simulink model "tempest_bpsk"  (R2018b)
settings: Solver=FixedStepDiscrete  StartTime=0.0  StopTime=inf  RelTol=1e-3
undefined symbols (not defined in the file): designMultirateFIR
libraries: commrfcorlib x2, commsync2 x2, commsdrhw_v2 x1, dspmlti4 x1, dspsigops x1, commrflib2 x1, commfilt2 x1
settings Model: SimulationMode=accelerator  Creator=Joseph  LastModifiedBy=Joseph

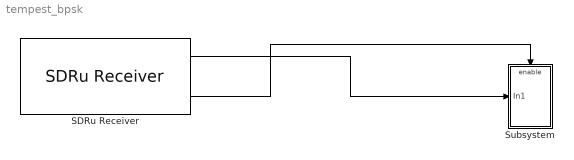
== system tempest_bpsk ==
  SDRu Receiver : commsdrhw_v2/SDRu Receiver  rxtx=rx  initializeIPAddress=0  devMap=0  USRP2_IP=192.168.10.2  USRP_IP_X300=192.168.10.2  USRP_IP_X310=192.168.10.2  USRP_serialNumB200=No devices found  USRP_serialNumB210=No devices found  platform=N200/N210/USRP2  prevPlatform=N200/N210/USRP2  lastIPAddressPopup=192.168.10.2  USRP_ID=192.168.10.2  LastIPAddress=192.168.10.2  ChannelMapping=1  centerFrequencySrc=Dialog  centerFrequency=54000000  loOffsetSrc=Dialog  loOffset=0  gainSrc=Dialog  gain=32  PPSSource=Internal  clockSource=Internal  masterClkRateParam=100e6  masterClkRateB200=32e6  masterClkRateB210=32e6  masterClkRateX300=200e6  masterClkRateX310=200e6  masterClkRate=100e6  decimInterpSrc=Dialog  decimInterp=512  USRP2_IP_NUM=[49 57 50 46 49 54 56 46 49 48 46 50]  TransportDataType=int16  overrunUnderrunPort=off  sampleTime=512/100e6  outputDatatype=double  frameLength=25472  HOST_DATA_PORT=0  HOST_CONTROL_PORT=0  USRP2_DATA_PORT=0  USRP2_CONTROL_PORT=0  bufferMode=Continuous streaming  EnableBurstMode=off  NumFramesInBurst=100
      settings: SourceProductName=Communications System Toolbox Support Package for USRP(R) Radio  SourceProductBaseCode=USRP
  Subsystem : Subsystem
  wires:
  SDRu Receiver/1 -> Subsystem/1(In1)
  SDRu Receiver/2 -> Subsystem/Enable

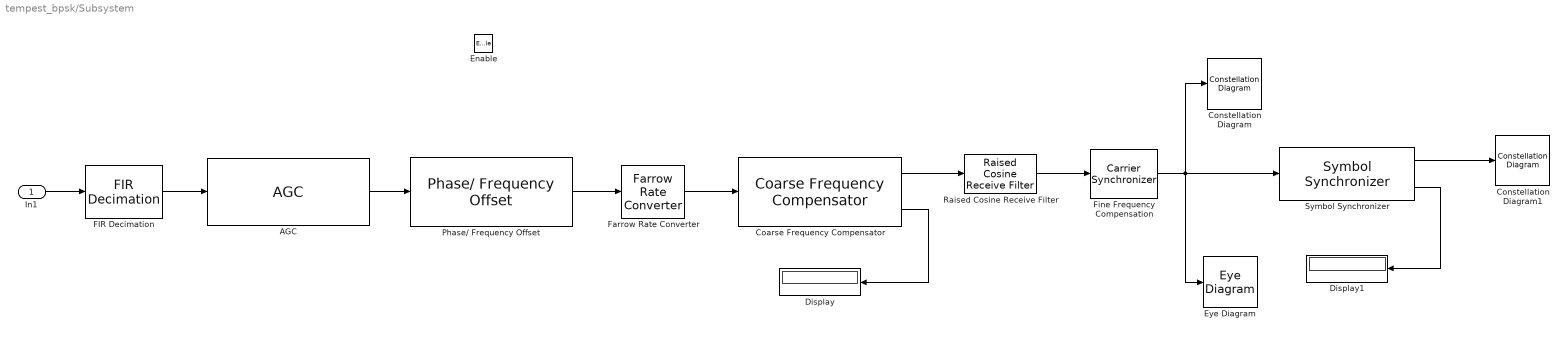
== system tempest_bpsk/Subsystem ==
  In1 : Inport
  Enable : EnablePort  PropagateVarSize=During execution
  AGC : commrfcorlib/AGC  LegacyMode=off  DetectorMethod=Rectifier  LoopMethod=Linear  UpdatePeriod=100  StepSize=0.1  AdaptationStepSize=0.01  DesiredOutputPower=1  AveragingLength=100  MaximumGain=30  MaxPowerGain=60  GainOutputPort=off  InputPowerOutputPort=off  SimulateUsing=Interpreted execution
      settings: SourceProductName=Communications System Toolbox
  Coarse Frequency Compensator : commrfcorlib/Coarse Frequency Compensator  Modulation=BPSK  Algorithm=FFT-based  FrequencyResolution=16  MaximumFrequencyOffset=3000  SamplesPerSymbol=4  EstimatedFreqOffsetPort=on  SimulateUsing=Code generation
      settings: SourceProductName=Communications System Toolbox  SourceProductBaseCode=CM
  Constellation Diagram : ConstellationDiagram
  Constellation Diagram1 : ConstellationDiagram
  Display : Display
      settings: Decimation=200
  Display1 : Display
      settings: Decimation=200
  Eye Diagram : EyeDiagram
  FIR Decimation : dspmlti4/FIR Decimation  FilterSource=Auto  h=designMultirateFIR(1,2)  D=16  filtStruct=Direct form  FilterObject=FDECIM  InputProcessing=Columns as channels (frame based)  framing=Enforce single-rate processing  inputOffset=0  outputBufInitCond=0  roundingMode=Floor  overflowMode=off  firstCoeffDataTypeStr=Inherit: Same word length as input  firstCoeffMin=[]  firstCoeffMax=[]  firstCoeffLastDataTypeStr=Inherit: Same word length as input  outputDataTypeStr=Inherit: Same as accumulator  outputMin=[]  outputMax=[]  outputLastDataTypeStr=Inherit: Same as accumulator
  Farrow Rate Converter : dspsigops/Farrow Rate Converter  InputSampleRate=100e6/512/16  OutputSampleRate=12000  OutputRateTolerance=0  Specification=Polynomial order  PolynomialOrder=4  Coefficients=[ -1, 1; 1, 0 ]  SimulateUsing=Code generation  roundingMode=Floor  overflowMode=off  CoefficientsDataTypeStr=fixdt(1,16)  FractionalDelayDataTypeStr=fixdt(0,8)  MultiplicandDataTypeStr=fixdt(1,16,13)  OutputDataTypeStr=Inherit: Same word length as input  OutputMin=[]  OutputMax=[]
      settings: SourceProductName=DSP System Toolbox  SourceProductBaseCode=DS
  Fine Frequency Compensation : commsync2/Carrier Synchronizer  Modulation=BPSK  ModulationPhaseOffset=Auto  CustomPhaseOffset=0  SamplesPerSymbol=200  DampingFactor=0.707  NormalizedLoopBandwidth=0.01  EstimatedPhaseErrorOutputPort=off  SimulateUsing=Code generation
      settings: SourceProductName=Communications Toolbox
  Phase/ Frequency Offset : commrflib2/Phase// Frequency Offset  phaseOffset=0  freqPort=off  freqOffset=-2400
      settings: SourceProductName=Communications System Toolbox
  Raised Cosine Receive Filter : commfilt2/Raised Cosine Receive Filter  filtType=Square root  R=0.5  filtSpan=4  N=200  downFactor=1  downOffset=0  filterGain=1  InputProcessing=Columns as channels (frame based)  RateOptions=Enforce single-rate processing  framing=Mute  checkCoeff=off  variableName=rcRxFilt  currentFiltSpan=4  D=(4)/2  inputOffset=0  sampMode=Mute  saveAsFlag=0  rateMode=Downsampling  checkGain=Normalized  launchFVT=on  roundingMode=Floor  overflowMode=off  coeffDataTypeStr=Inherit: Same word length as input  coeffMin=[]  coeffMax=[]  coeffLastDataTypeStr=Inherit: Same word length as input  accumDataTypeStr=Inherit: Same as product output  accumLastDataTypeStr=Inherit: Same as product output  outputDataTypeStr=Inherit: Same as accumulator  outputMin=[]  outputMax=[]  outputLastDataTypeStr=Inherit: Same as accumulator
      settings: SourceProductName=Communications Toolbox
  Symbol Synchronizer : commsync2/Symbol Synchronizer  Modulation=PAM/PSK/QAM  TimingErrorDetector=Gardner (non-data-aided)  SamplesPerSymbol=200  DampingFactor=1  NormalizedLoopBandwidth=0.005  DetectorGain=2.7  TimingErrorOutputPort=on  SimulateUsing=Code generation
      settings: SourceProductName=Communications System Toolbox  SourceProductBaseCode=CM
  wires:
  In1/1 -> FIR Decimation/1
  Farrow Rate Converter/1 -> Coarse Frequency Compensator/1
  FIR Decimation/1 -> AGC/1
  AGC/1 -> Phase/ Frequency Offset/1
  Phase/ Frequency Offset/1 -> Farrow Rate Converter/1
  Coarse Frequency Compensator/1 -> Raised Cosine Receive Filter/1
  Raised Cosine Receive Filter/1 -> Fine Frequency Compensation/1
  Coarse Frequency Compensator/2 -> Display/1
  Fine Frequency Compensation/1 -> Constellation Diagram/1, Symbol Synchronizer/1, Eye Diagram/1
  Symbol Synchronizer/1 -> Constellation Diagram1/1
  Symbol Synchronizer/2 -> Display1/1
